simulink model "suspension_simulink"  (R2024a)
settings: Solver=VariableStepAuto  StartTime=0.0  StopTime=10.0  RelTol=1e-3
values from neighbouring files (symbols this model uses):
  b1 = 1000    [dinamica_suspension.m]
  k1 = 16182    [dinamica_suspension.m]
  k2 = 19000    [dinamica_suspension.m]
  m1 = 290    [dinamica_suspension.m]
  m2 = 59    [dinamica_suspension.m]
settings Model: Creator=USUARIO  LastModifiedBy=USUARIO

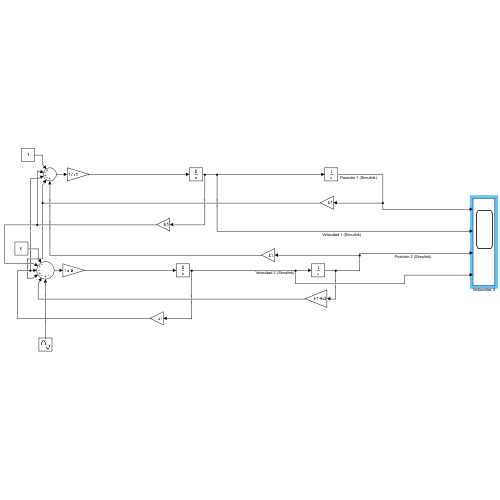
[thumbnail: Simulink's stored preview of the top-level diagram]
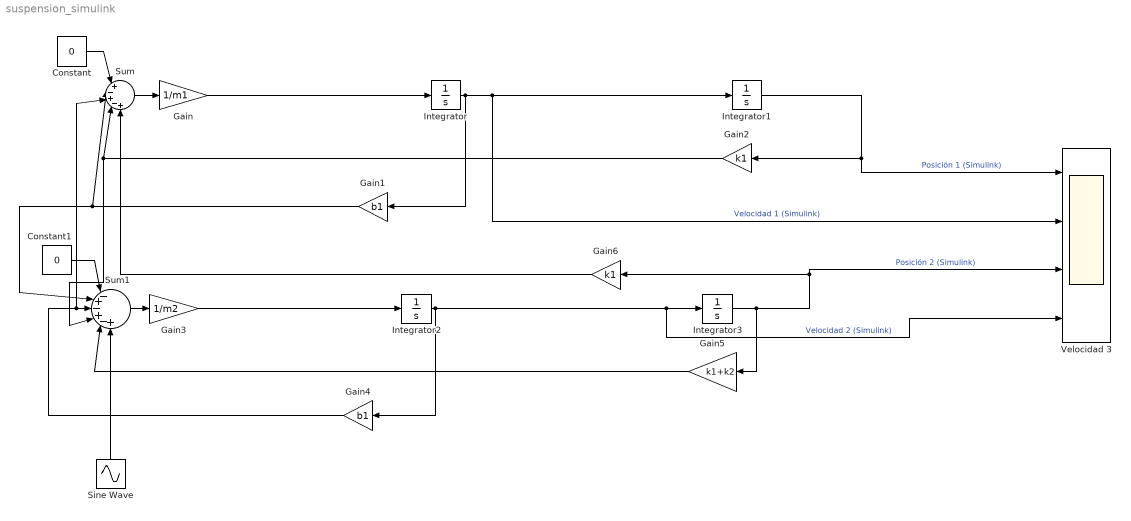
== system suspension_simulink ==
  Constant : Constant  Value=0
  Constant1 : Constant  Value=0
  Gain : Gain  Gain=1/m1
  Gain1 : Gain  Gain=b1
  Gain2 : Gain  Gain=k1
  Gain3 : Gain  Gain=1/m2
  Gain4 : Gain  Gain=b1
  Gain5 : Gain  Gain=k1+k2
  Gain6 : Gain  Gain=k1
  Integrator{,1..3} (4 alike) : Integrator
  Sine Wave : Sin  Amplitude=0.05*k2  Frequency=0.5*pi  SampleTime=0
  Sum : Sum  Inputs=|+-+-+
  Sum1 : Sum  Inputs=|-+-+-+
  Velocidad 3 : Scope  NumInputPorts=4
  wires:
  Constant1/1 -> Sum1/1
  Sum1/1 -> Gain3/1
  Sine Wave/1 -> Sum1/6
  Integrator2/1 -> Velocidad 3/4, Integrator3/1, Gain4/1  "Velocidad 2 (Simulink)"
  Gain/1 -> Integrator/1
  Gain6/1 -> Sum/5
  Gain3/1 -> Integrator2/1
  Gain4/1 -> Sum/3, Sum1/3
  Integrator3/1 -> Velocidad 3/3, Gain6/1, Gain5/1  "Posición 2 (Simulink)"
  Gain2/1 -> Sum1/4, Sum/4
  Constant/1 -> Sum/1
  Integrator1/1 -> Velocidad 3/1, Gain2/1  "Posición 1 (Simulink)"
  Gain1/1 -> Sum1/2, Sum/2
  Integrator/1 -> Gain1/1, Velocidad 3/2, Integrator1/1  "Velocidad 1 (Simulink)"
  Gain5/1 -> Sum1/5
  Sum/1 -> Gain/1
